simulink model "model5_2_k"  (R2024b)
settings: Solver=FixedStepAuto  StartTime=0.0  StopTime=15  FixedStep=0.0001  RelTol=1e-3
values from neighbouring files (symbols this model uses):
  Rk = [1, RS(1)', 0]    [domaci5.m]    (also in domaci5_2_k.m = [1, RS(1), w^2, w^2 * RS(1)])
  Sk = RS(2:end)'    [domaci5.m]    (also in domaci5_2_k.m)
  Tsk = 1 / dcgain(1/Rsk * feedback(Gpk, Ssk/Rsk))    [domaci5_2_k.m]
  w = 2    [domaci5_2_k.m]
settings Model: Creator=neso  LastModifiedBy=neso

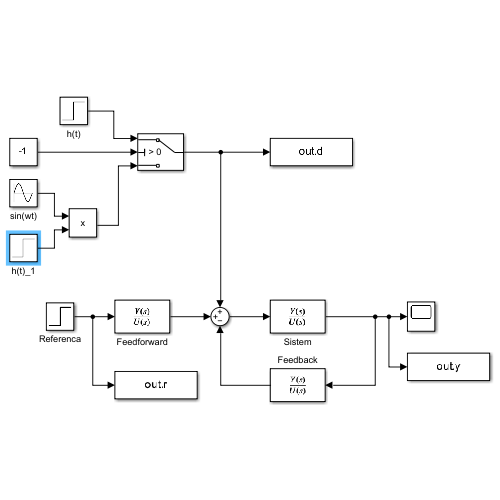
[thumbnail: Simulink's stored preview of the top-level diagram]
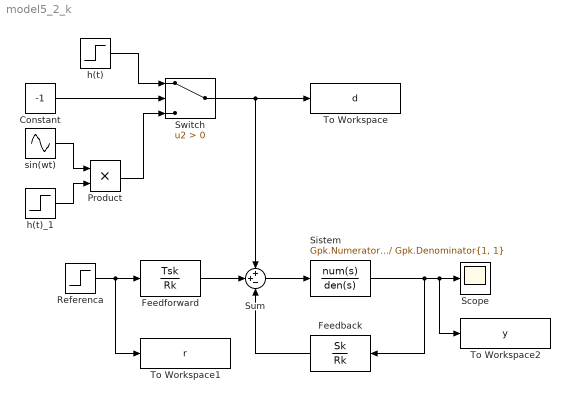
== system model5_2_k ==
  Constant : Constant  Value=-1
  Feedback : TransferFcn  Numerator=Sk  Denominator=Rk
  Feedforward : TransferFcn  Numerator=Tsk  Denominator=Rk
  Product : Product
  Referenca : Step  Time=0  After=5  SampleTime=0
  Scope : Scope
  Sistem : TransferFcn  Numerator=Gpk.Numerator{1, 1}  Denominator=Gpk.Denominator{1, 1}
  Sum : Sum  Inputs=++-
  Switch : Switch  Criteria=u2 > Threshold  SaturateOnIntegerOverflow=off  InputSameDT=off
  To Workspace : ToWorkspace  VariableName=d  SaveFormat=Timeseries  SampleTime=-1
  To Workspace1 : ToWorkspace  VariableName=r  SaveFormat=Timeseries  SampleTime=-1
  To Workspace2 : ToWorkspace  VariableName=y  SaveFormat=Timeseries  SampleTime=-1
  h(t) : Step  Time=5  After=2  SampleTime=0
  h(t)_1 : Step  Time=5  SampleTime=0
  sin(wt) : Sin  Frequency=w  SampleTime=0
  wires:
  Sum/1 -> Sistem/1
  Feedforward/1 -> Sum/2
  Referenca/1 -> To Workspace1/1, Feedforward/1
  Feedback/1 -> Sum/3
  Sistem/1 -> To Workspace2/1, Scope/1, Feedback/1
  h(t)/1 -> Switch/1
  Switch/1 -> To Workspace/1, Sum/1
  Constant/1 -> Switch/2
  Product/1 -> Switch/3
  sin(wt)/1 -> Product/1
  h(t)_1/1 -> Product/2
